simulink model "SchematJK"  (R2018b)
settings: Solver=VariableStepAuto  StartTime=0.0  StopTime=10.0  RelTol=1e-3
libraries: simulink_extras x2
settings Model: Creator=bartl  LastModifiedBy=bartl

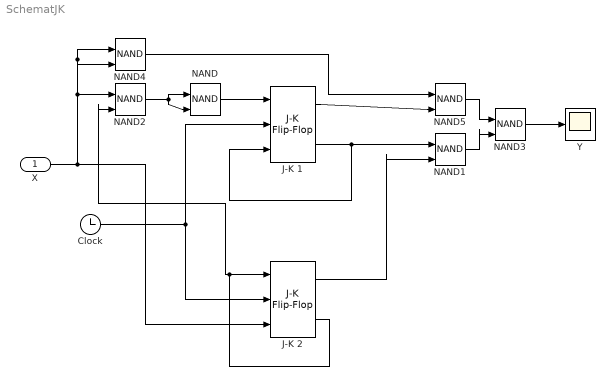
== system SchematJK ==
  X : Inport
  Clock : Clock
  J-K 1 : simulink_extras/Flip Flops/J-K Flip-Flop  initial_condition=0
      settings: SourceProductName=Simulink
  J-K 2 : simulink_extras/Flip Flops/J-K Flip-Flop  initial_condition=0
      settings: SourceProductName=Simulink
  NAND{,1..5} (6 alike) : Logic  Operator=NAND  IconShape=distinctive  AllPortsSameDT=off  OutDataTypeStr=boolean
  Y : Scope
  wires:
  Clock/1 -> J-K 1/2, J-K 2/2
  X/1 -> J-K 2/3, NAND4/1, NAND4/2, NAND2/1
  J-K 1/2 -> J-K 1/3, NAND1/1
  J-K 2/2 -> NAND2/2, J-K 2/1
  NAND/1 -> J-K 1/1
  NAND2/1 -> NAND/2, NAND/1
  J-K 2/1 -> NAND1/2
  J-K 1/1 -> NAND5/2
  NAND4/1 -> NAND5/1
  NAND1/1 -> NAND3/2
  NAND5/1 -> NAND3/1
  NAND3/1 -> Y/1
